simulink model "ANN_and_Fuzzy_NCD"  (R2024a)
settings: Solver=ode23  StartTime=0.0  StopTime=200  RelTol=1e-8  EnableMultiTasking=on
model workspace (MAT data in the model file):
  targetSettings3 : object (value not decoded)
values from neighbouring files (symbols this model uses):
  I = in1'    [ann_training.m]
  T = out1'    [ann_training.m]
undefined symbols (not defined in the file or in its folder): B, DL, DQ, m, M, magnitude, rg, W, xb, xg, Xudot, yb, yg, Yvdot, zb, zg, Zwdot
libraries: neural x270, simulink x28, fuzblock x3
(part 11 of 12)

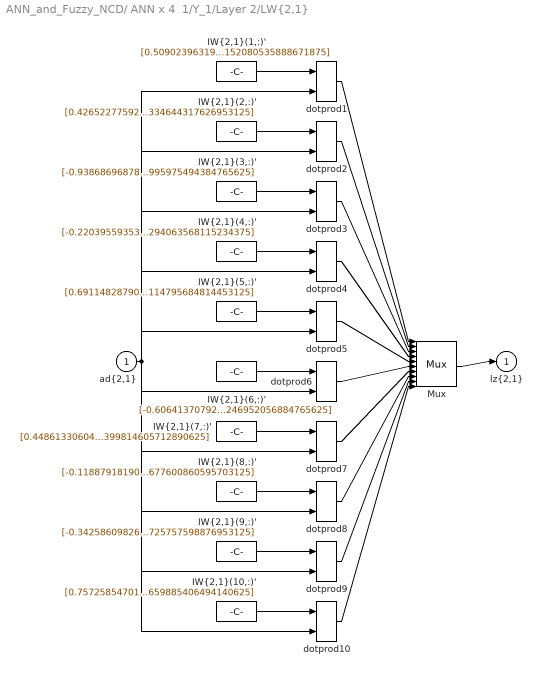
== system ANN_and_Fuzzy_NCD/ ANN x 4  1/Y_1/Layer 2/LW{2,1} ==
  "ad{2,1}" : Inport  PortDimensions=20
      mask Display: e = 0.06;c1 = [120 230 180]/255;c2 = ([120 230 180]+0)/(256+128);c3 = ([120 230 180]+128)/(256+128);patch([0 1 1 0],[0 0 1 1],c1);patch([0 1 1 1-e 1-e 0+e],[0 0 1 1-e 0+e 0+e],c2);patch([0 0 1 1-e 0+e 0+e],[0 1 1 1-e 1-e 0+e],c3);plot([0 1 1 0 0],[0 0 1 1 0]);
  "IW{2,1}(1,:)'" : Constant  Value=[0.5090239631979407430861783723230473697185516357421875;0.11160391846070348564889940234934329055249691009521484375;-0.60838467523272410364398865567636676132678985595703125;-0.45293416178246503900339803294627927243709564208984375;0.311166634755049076321853362969704903662204742431640625;0.330355832861899789687498696366674266755580902099609375;-0.57422288061641513223776200902648270130157470703125;-0.2838835075137227104136172783910296857357025146484375;-0.428001029373137054090392439320567063987255096435546875;0.62000342652741713411757018548087216913700103759765625;0.74336850402159060369200460627325810492038726806640625;-0.01139508661315961901561166769170085899531841278076171875;-0.61400475923319619564466620431630872189998626708984375;-0.05991076251349496117892812208083341829478740692138671875;0.84943975721566922221228423950378783047199249267578125;0.558146672456232284531552068074233829975128173828125;-0.042015831108889532818917444956241524778306484222412109375;0.460089284343286164524755577076575718820095062255859375;0.1646087842077264273843439923439291305840015411376953125;1.066820046479761696645027768681757152080535888671875]
      mask Display: e = 0.06;c1 = [120 150 230]/255;c2 = ([120 150 230]+0)/383;c3 = ([120 150 230]+128)/383;patch([0 1 1 0],[0 0 1 1],c1);patch([0 1 1 1-e 1-e 0+e],[0 0 1 1-e 0+e 0+e],c2);patch([0 0 1 1-e 0+e 0+e],[0 1 1 1-e 1-e 0+e],c3);plot([0 1 1 0 0],[0 0 1 1 0]);disp('weights');
  "IW{2,1}(10,:)'" : Constant  Value=[0.75725854701721961870219956836081109941005706787109375;0.74786484659251584172778848369489423930644989013671875;-0.37330720116505722305788594894693233072757720947265625;-0.25560543970363325261274667354882694780826568603515625;-0.3955234726214145180023251668899320065975189208984375;-0.1170710839775310485588732944961520843207836151123046875;0.130515477526785550477228525778627954423427581787109375;0.2277678588107421575603694918754626996815204620361328125;0.33980433602491155742342243684106506407260894775390625;-0.5489951844676215220175663489499129354953765869140625;0.7317112584413199005695105370250530540943145751953125;-0.42224791132812555805031706768204458057880401611328125;-0.11131793040447192366659834306119591929018497467041015625;-0.24585736991511353277672924377839080989360809326171875;-0.5961164816487041218096010197768919169902801513671875;-0.03003556254240373479813541734984028153121471405029296875;0.08420958263756218864504177190610789693892002105712890625;0.9050366596150227760375628349720500409603118896484375;0.46753348003908323793353929431759752333164215087890625;-0.039178527082161240802093971069552935659885406494140625]
      mask Display: e = 0.06;c1 = [120 150 230]/255;c2 = ([120 150 230]+0)/383;c3 = ([120 150 230]+128)/383;patch([0 1 1 0],[0 0 1 1],c1);patch([0 1 1 1-e 1-e 0+e],[0 0 1 1-e 0+e 0+e],c2);patch([0 0 1 1-e 0+e 0+e],[0 1 1 1-e 1-e 0+e],c3);plot([0 1 1 0 0],[0 0 1 1 0]);disp('weights');
  "IW{2,1}(2,:)'" : Constant  Value=[0.426522775921342967020422065616003237664699554443359375;0.11669002064379037364449942515420843847095966339111328125;-0.09094231709906390459519087698936345987021923065185546875;0.567514248708034241275299791595898568630218505859375;0.2537304330577907496291345523786731064319610595703125;-1.2920604784385449903538756188936531543731689453125;0.3414812039848078573101020083413459360599517822265625;0.263963170000102831380672796512953937053680419921875;-1.09849856655470023980569749255664646625518798828125;0.9864726214973646989392364048399031162261962890625;0.003132022306092559216228465857057017274200916290283203125;0.31270444346332448848357898896210826933383941650390625;-0.25315824125565578039953607003553770482540130615234375;-0.69773460760423111626238323879078961908817291259765625;-0.07611461049244357124354820598455262370407581329345703125;0.89021133988713707640982875091140158474445343017578125;0.6226655353392629432818239365587942302227020263671875;0.59260455755274688005584948768955655395984649658203125;-0.409387777619778514548443126841448247432708740234375;0.5890538696326192980023961354163475334644317626953125]
      mask Display: e = 0.06;c1 = [120 150 230]/255;c2 = ([120 150 230]+0)/383;c3 = ([120 150 230]+128)/383;patch([0 1 1 0],[0 0 1 1],c1);patch([0 1 1 1-e 1-e 0+e],[0 0 1 1-e 0+e 0+e],c2);patch([0 0 1 1-e 0+e 0+e],[0 1 1 1-e 1-e 0+e],c3);plot([0 1 1 0 0],[0 0 1 1 0]);disp('weights');
  "IW{2,1}(3,:)'" : Constant  Value=[-0.93868696878192781074545791852870024740695953369140625;-0.6377553662566040060255545540712773799896240234375;0.86418031487382329647317646958981640636920928955078125;1.0260293267344493539638961010496132075786590576171875;-0.58952068410571223378013883120729587972164154052734375;0.0992184017356094738460114967892877757549285888671875;0.62408971093074072644668603970785625278949737548828125;0.1697386682494127219111845761290169321000576019287109375;-1.1731596069625862543972516505164094269275665283203125;0.76298716435795699286614990342059172689914703369140625;-0.24277211963838796204839809433906339108943939208984375;-1.197372360644966438059100255486555397510528564453125;0.0712172363293012422591488075340748764574527740478515625;0.631562196722546875804482624516822397708892822265625;-0.192844601384166980384549106020131148397922515869140625;-0.1418385019727086138185967456593061797320842742919921875;0.386434553732358854194472996823606081306934356689453125;0.883931218735329427005353863933123648166656494140625;0.83856934978820907300445242071873508393764495849609375;1.8159130409844428388765891213552094995975494384765625]
      mask Display: e = 0.06;c1 = [120 150 230]/255;c2 = ([120 150 230]+0)/383;c3 = ([120 150 230]+128)/383;patch([0 1 1 0],[0 0 1 1],c1);patch([0 1 1 1-e 1-e 0+e],[0 0 1 1-e 0+e 0+e],c2);patch([0 0 1 1-e 0+e 0+e],[0 1 1 1-e 1-e 0+e],c3);plot([0 1 1 0 0],[0 0 1 1 0]);disp('weights');
  "IW{2,1}(4,:)'" : Constant  Value=[-0.22039559353873261482448242531972937285900115966796875;-0.2045148569053286402574798330533667467534542083740234375;-0.486566430678849914936989762281882576644420623779296875;-0.07025821021501608976134178874417557381093502044677734375;-0.658874386397240385804252582602202892303466796875;0.269798175500027159756655237288214266300201416015625;-0.1315210626537921811962661422512610442936420440673828125;-0.50169234000809359574901691303239203989505767822265625;2.141580948732917821786259082728065550327301025390625;0.37679791717396271533147000809549354016780853271484375;0.30916188174127656740353131681331433355808258056640625;-0.767499015164006426203968658228404819965362548828125;0.8980414488971601993938520536175929009914398193359375;-0.63991664257674429894251488804002292454242706298828125;-0.54821013988044364761975657529546879231929779052734375;0.52885732193772228004746693841298110783100128173828125;0.1540261738452853579328660771352588199079036712646484375;0.01847479725367588698770049404629389755427837371826171875;-0.333797443500849888575743307228549383580684661865234375;0.026821807331764944970498021348248585127294063568115234375]
      mask Display: e = 0.06;c1 = [120 150 230]/255;c2 = ([120 150 230]+0)/383;c3 = ([120 150 230]+128)/383;patch([0 1 1 0],[0 0 1 1],c1);patch([0 1 1 1-e 1-e 0+e],[0 0 1 1-e 0+e 0+e],c2);patch([0 0 1 1-e 0+e 0+e],[0 1 1 1-e 1-e 0+e],c3);plot([0 1 1 0 0],[0 0 1 1 0]);disp('weights');
  "IW{2,1}(5,:)'" : Constant  Value=[0.69114828790033266958658941803150810301303863525390625;0.55435534445943213111007707993849180638790130615234375;-0.9176208324668231330889511809800751507282257080078125;-0.10491305465673463059861347801415831781923770904541015625;-0.05473083756133391430953594181119115091860294342041015625;-0.27525707289210676886881401514983735978603363037109375;-0.0745176702560048642709489286062307655811309814453125;0.7894568146855700518926823860965669155120849609375;-1.68541642068066277460047786007635295391082763671875;-0.314903937294579494565738286837586201727390289306640625;0.1435542443257350198049238088060519658029079437255859375;-0.01012709573370276262826994440047201351262629032135009765625;0.16378713151763435451613304394413717091083526611328125;-0.361346282484408087842808754430734552443027496337890625;-0.03471757844671798098890036499142297543585300445556640625;-0.1938551744629932738206434805761091411113739013671875;-1.0324162610677387608149047082406468689441680908203125;-0.363503597064038341812874932656995952129364013671875;-0.4326961798445900786447282371227629482746124267578125;-0.65375618486997399969595790025778114795684814453125]
      mask Display: e = 0.06;c1 = [120 150 230]/255;c2 = ([120 150 230]+0)/383;c3 = ([120 150 230]+128)/383;patch([0 1 1 0],[0 0 1 1],c1);patch([0 1 1 1-e 1-e 0+e],[0 0 1 1-e 0+e 0+e],c2);patch([0 0 1 1-e 0+e 0+e],[0 1 1 1-e 1-e 0+e],c3);plot([0 1 1 0 0],[0 0 1 1 0]);disp('weights');
  "IW{2,1}(6,:)'" : Constant  Value=[-0.6064137079235631944129636394791305065155029296875;-0.70430664427252132053780542264576070010662078857421875;1.128267088531079931357226087129674851894378662109375;-0.01443760284603235431732937144033712684176862239837646484375;-0.1665820411319823557416697212829603813588619232177734375;-0.5448969322325221131819716902100481092929840087890625;0.1500632983600085623709929905089666135609149932861328125;0.491239762856461814610753435772494412958621978759765625;1.34531361537262217353827509214170277118682861328125;-0.65877809908486562040508260906790383160114288330078125;-0.2179297474681796409345935217061196453869342803955078125;-0.33324003089934317589637657874845899641513824462890625;0.331240335532091478842886544953216798603534698486328125;-0.140788452060973512391939266308327205479145050048828125;0.470179717315354850359909733015228994190692901611328125;0.32670818751247054922970391999115236103534698486328125;-0.30544754941956397953362056796322576701641082763671875;-0.179740446791701480311331806660746224224567413330078125;-0.53222231123358465509909365209750831127166748046875;-0.4198763573104165036653512288467027246952056884765625]
      mask Display: e = 0.06;c1 = [120 150 230]/255;c2 = ([120 150 230]+0)/383;c3 = ([120 150 230]+128)/383;patch([0 1 1 0],[0 0 1 1],c1);patch([0 1 1 1-e 1-e 0+e],[0 0 1 1-e 0+e 0+e],c2);patch([0 0 1 1-e 0+e 0+e],[0 1 1 1-e 1-e 0+e],c3);plot([0 1 1 0 0],[0 0 1 1 0]);disp('weights');
  "IW{2,1}(7,:)'" : Constant  Value=[0.448613306043071202733329982947907410562038421630859375;-0.1822903414610920480587452630061306990683078765869140625;-0.2126563507677423359165658212077687494456768035888671875;-0.28907878885491478104796669867937453091144561767578125;-0.5546330576663585087970886888797394931316375732421875;0.0881391364579335034878937449320801533758640289306640625;-0.005256269492573631234300091108480046386830508708953857421875;-0.13134253211367508118456726151634939014911651611328125;0.07828790111291732134457532765736686997115612030029296875;0.17303125336206737205912986610201187431812286376953125;0.04399549925057953669860211221021017991006374359130859375;0.1570358748639592849638546567803132347762584686279296875;-0.17807543738489750584363946472876705229282379150390625;0.2247661710889533315249622091869241558015346527099609375;-0.10691750616299990073176928717657574452459812164306640625;0.10221326745057923712778347180574201047420501708984375;0.94604303586329352437900297445594333112239837646484375;-0.31025843146322407140047516804770566523075103759765625;0.35028098540476559907830278461915440857410430908203125;-0.039186964941104164561469502814361476339399814605712890625]
      mask Display: e = 0.06;c1 = [120 150 230]/255;c2 = ([120 150 230]+0)/383;c3 = ([120 150 230]+128)/383;patch([0 1 1 0],[0 0 1 1],c1);patch([0 1 1 1-e 1-e 0+e],[0 0 1 1-e 0+e 0+e],c2);patch([0 0 1 1-e 0+e 0+e],[0 1 1 1-e 1-e 0+e],c3);plot([0 1 1 0 0],[0 0 1 1 0]);disp('weights');
  "IW{2,1}(8,:)'" : Constant  Value=[-0.1188791819001266680810857678807224147021770477294921875;-0.5328985881442112049199977263924665749073028564453125;0.5259930043630609564075939488247968256473541259765625;-0.355545136520511118050080767716281116008758544921875;-0.436040224271254495125305084002320654690265655517578125;-0.38339149391564586455416474564117379486560821533203125;-0.485397555278109849030698796923388727009296417236328125;-0.53377520344499862492426700555370189249515533447265625;1.538462588979844003489461101708002388477325439453125;0.240654646945936523394493633531965315341949462890625;0.65460238834859796330789549756445921957492828369140625;0.216226396066736936685259706791839562356472015380859375;-0.284211662449685931175480391175369732081890106201171875;-0.41705775992225502246668611405766569077968597412109375;-0.56091006758118755470832184073515236377716064453125;-0.6274337920918444666540381149388849735260009765625;1.057837377776273957152852744911797344684600830078125;-0.425439205099200690174399142051697708666324615478515625;-0.341212462205700839401600887867971323430538177490234375;0.0115945042058083098990284298679398489184677600860595703125]
      mask Display: e = 0.06;c1 = [120 150 230]/255;c2 = ([120 150 230]+0)/383;c3 = ([120 150 230]+128)/383;patch([0 1 1 0],[0 0 1 1],c1);patch([0 1 1 1-e 1-e 0+e],[0 0 1 1-e 0+e 0+e],c2);patch([0 0 1 1-e 0+e 0+e],[0 1 1 1-e 1-e 0+e],c3);plot([0 1 1 0 0],[0 0 1 1 0]);disp('weights');
  "IW{2,1}(9,:)'" : Constant  Value=[-0.3425860982600339443848724840790964663028717041015625;0.317963370391335209408367745709256269037723541259765625;0.38600757975739430349904068862088024616241455078125;0.11942370995519570320286817377564148046076297760009765625;-0.135297761504829860967902277479879558086395263671875;0.3811740311196782915459380092215724289417266845703125;-0.09833512570032722222013177315602661110460758209228515625;0.09431607025873588179276651999316527508199214935302734375;0.108063697459556851132589372355141676962375640869140625;0.93226980443745766091723226054455153644084930419921875;-0.198985445557301410257622364952112548053264617919921875;0.07278341181556084726889110925185377709567546844482421875;0.66596047086168541628836692325421608984470367431640625;-0.27925246224251842885877294975216500461101531982421875;-0.31408901001109590378490565854008309543132781982421875;-0.70192808772125558913757004120270721614360809326171875;-1.3726680003553408671024271825444884598255157470703125;-0.7352673542920313831672274318407289683818817138671875;-0.2476548671200008711057449772852123714983463287353515625;1.0455333746920534299107430342701263725757598876953125]
      mask Display: e = 0.06;c1 = [120 150 230]/255;c2 = ([120 150 230]+0)/383;c3 = ([120 150 230]+128)/383;patch([0 1 1 0],[0 0 1 1],c1);patch([0 1 1 1-e 1-e 0+e],[0 0 1 1-e 0+e 0+e],c2);patch([0 0 1 1-e 0+e 0+e],[0 1 1 1-e 1-e 0+e],c3);plot([0 1 1 0 0],[0 0 1 1 0]);disp('weights');
  Mux : Mux  Inputs=10
      mask Display: e = 0.06;c1 = [120 150 230]/255;c2 = ([120 150 230]+0)/383;c3 = ([120 150 230]+128)/383;patch([0 1 1 0],[0 0 1 1],c1);patch([0 1 1 1-e 1-e 0+e],[0 0 1 1-e 0+e 0+e],c2);patch([0 0 1 1-e 0+e 0+e],[0 1 1 1-e 1-e 0+e],c3);plot([0 1 1 0 0],[0 0 1 1 0]);disp('Mux');
  dotprod{1..10} (10 alike) : neural/Weight Functions/dotprod
  "lz{2,1}" : Outport
      mask Display: e = 0.06;c1 = [120 230 180]/255;c2 = ([120 230 180]+0)/(256+128);c3 = ([120 230 180]+128)/(256+128);patch([0 1 1 0],[0 0 1 1],c1);patch([0 1 1 1-e 1-e 0+e],[0 0 1 1-e 0+e 0+e],c2);patch([0 0 1 1-e 0+e 0+e],[0 1 1 1-e 1-e 0+e],c3);plot([0 1 1 0 0],[0 0 1 1 0]);
  wires:
  "IW{2,1}(1,:)'"/1 -> dotprod1/1
  "ad{2,1}"/1 -> dotprod1/2, dotprod2/2, dotprod3/2, dotprod4/2, dotprod5/2, dotprod6/2, dotprod7/2, dotprod8/2, dotprod9/2, dotprod10/2
  dotprod1/1 -> Mux/1
  "IW{2,1}(2,:)'"/1 -> dotprod2/1
  dotprod2/1 -> Mux/2
  "IW{2,1}(3,:)'"/1 -> dotprod3/1
  dotprod3/1 -> Mux/3
  "IW{2,1}(4,:)'"/1 -> dotprod4/1
  dotprod4/1 -> Mux/4
  "IW{2,1}(5,:)'"/1 -> dotprod5/1
  dotprod5/1 -> Mux/5
  "IW{2,1}(6,:)'"/1 -> dotprod6/1
  dotprod6/1 -> Mux/6
  "IW{2,1}(7,:)'"/1 -> dotprod7/1
  dotprod7/1 -> Mux/7
  "IW{2,1}(8,:)'"/1 -> dotprod8/1
  dotprod8/1 -> Mux/8
  "IW{2,1}(9,:)'"/1 -> dotprod9/1
  dotprod9/1 -> Mux/9
  "IW{2,1}(10,:)'"/1 -> dotprod10/1
  dotprod10/1 -> Mux/10
  Mux/1 -> "lz{2,1}"/1

== system ANN_and_Fuzzy_NCD/ ANN x 4  1/Y_1/Layer 3/Delays 1 ==
  "p{3}" : Inport  PortDimensions=10
      mask Display: e = 0.06;c1 = [120 230 180]/255;c2 = ([120 230 180]+0)/(256+128);c3 = ([120 230 180]+128)/(256+128);patch([0 1 1 0],[0 0 1 1],c1);patch([0 1 1 1-e 1-e 0+e],[0 0 1 1-e 0+e 0+e],c2);patch([0 0 1 1-e 0+e 0+e],[0 1 1 1-e 1-e 0+e],c3);plot([0 1 1 0 0],[0 0 1 1 0]);
  mux : Mux  Inputs=1
      mask Display: e = 0.06;c1 = [120 150 230]/255;c2 = ([120 150 230]+0)/383;c3 = ([120 150 230]+128)/383;patch([0 1 1 0],[0 0 1 1],c1);patch([0 1 1 1-e 1-e 0+e],[0 0 1 1-e 0+e 0+e],c2);patch([0 0 1 1-e 0+e 0+e],[0 1 1 1-e 1-e 0+e],c3);plot([0 1 1 0 0],[0 0 1 1 0]);disp('Mux')
  "pd{3,2}" : Outport
      mask Display: e = 0.06;c1 = [120 230 180]/255;c2 = ([120 230 180]+0)/(256+128);c3 = ([120 230 180]+128)/(256+128);patch([0 1 1 0],[0 0 1 1],c1);patch([0 1 1 1-e 1-e 0+e],[0 0 1 1-e 0+e 0+e],c2);patch([0 0 1 1-e 0+e 0+e],[0 1 1 1-e 1-e 0+e],c3);plot([0 1 1 0 0],[0 0 1 1 0]);
  wires:
  "p{3}"/1 -> mux/1
  mux/1 -> "pd{3,2}"/1

== system ANN_and_Fuzzy_NCD/ ANN x 4  1/Y_1/Layer 3/LW{3,2} ==
  "ad{3,2}" : Inport  PortDimensions=10
      mask Display: e = 0.06;c1 = [120 230 180]/255;c2 = ([120 230 180]+0)/(256+128);c3 = ([120 230 180]+128)/(256+128);patch([0 1 1 0],[0 0 1 1],c1);patch([0 1 1 1-e 1-e 0+e],[0 0 1 1-e 0+e 0+e],c2);patch([0 0 1 1-e 0+e 0+e],[0 1 1 1-e 1-e 0+e],c3);plot([0 1 1 0 0],[0 0 1 1 0]);
  "IW{3,2}(1,:)'" : Constant  Value=[-0.112703050539125104734239357640035450458526611328125;0.0026845090711100434884006649127741184202022850513458251953125;-0.006133432667343429074702232384197486680932343006134033203125;0.1331845640688972542964307876900420524179935455322265625;0.0978135232567727275210245352354831993579864501953125;0.71146262583635844212182064438820816576480865478515625;-0.151075401259040287271773195243440568447113037109375;0.11540184957138906185480919930341769941151142120361328125;0.07846874545309991122454817968900897540152072906494140625;0.1909190666063294294918506466274266131222248077392578125]
      mask Display: e = 0.06;c1 = [120 150 230]/255;c2 = ([120 150 230]+0)/383;c3 = ([120 150 230]+128)/383;patch([0 1 1 0],[0 0 1 1],c1);patch([0 1 1 1-e 1-e 0+e],[0 0 1 1-e 0+e 0+e],c2);patch([0 0 1 1-e 0+e 0+e],[0 1 1 1-e 1-e 0+e],c3);plot([0 1 1 0 0],[0 0 1 1 0]);disp('weights');
  Mux : Mux  Inputs=1
      mask Display: e = 0.06;c1 = [120 150 230]/255;c2 = ([120 150 230]+0)/383;c3 = ([120 150 230]+128)/383;patch([0 1 1 0],[0 0 1 1],c1);patch([0 1 1 1-e 1-e 0+e],[0 0 1 1-e 0+e 0+e],c2);patch([0 0 1 1-e 0+e 0+e],[0 1 1 1-e 1-e 0+e],c3);plot([0 1 1 0 0],[0 0 1 1 0]);disp('Mux');
  dotprod1 : neural/Weight Functions/dotprod
  "lz{3,2}" : Outport
      mask Display: e = 0.06;c1 = [120 230 180]/255;c2 = ([120 230 180]+0)/(256+128);c3 = ([120 230 180]+128)/(256+128);patch([0 1 1 0],[0 0 1 1],c1);patch([0 1 1 1-e 1-e 0+e],[0 0 1 1-e 0+e 0+e],c2);patch([0 0 1 1-e 0+e 0+e],[0 1 1 1-e 1-e 0+e],c3);plot([0 1 1 0 0],[0 0 1 1 0]);
  wires:
  "IW{3,2}(1,:)'"/1 -> dotprod1/1
  "ad{3,2}"/1 -> dotprod1/2
  dotprod1/1 -> Mux/1
  Mux/1 -> "lz{3,2}"/1

== system ANN_and_Fuzzy_NCD/ ANN x 4  1/Z_1/Layer 1/Delays 1 ==
  "p{1}" : Inport  PortDimensions=2
      mask Display: e = 0.06;c1 = [120 230 180]/255;c2 = ([120 230 180]+0)/(256+128);c3 = ([120 230 180]+128)/(256+128);patch([0 1 1 0],[0 0 1 1],c1);patch([0 1 1 1-e 1-e 0+e],[0 0 1 1-e 0+e 0+e],c2);patch([0 0 1 1-e 0+e 0+e],[0 1 1 1-e 1-e 0+e],c3);plot([0 1 1 0 0],[0 0 1 1 0]);
  mux : Mux  Inputs=1
      mask Display: e = 0.06;c1 = [120 150 230]/255;c2 = ([120 150 230]+0)/383;c3 = ([120 150 230]+128)/383;patch([0 1 1 0],[0 0 1 1],c1);patch([0 1 1 1-e 1-e 0+e],[0 0 1 1-e 0+e 0+e],c2);patch([0 0 1 1-e 0+e 0+e],[0 1 1 1-e 1-e 0+e],c3);plot([0 1 1 0 0],[0 0 1 1 0]);disp('Mux')
  "pd{1,1}" : Outport
      mask Display: e = 0.06;c1 = [120 230 180]/255;c2 = ([120 230 180]+0)/(256+128);c3 = ([120 230 180]+128)/(256+128);patch([0 1 1 0],[0 0 1 1],c1);patch([0 1 1 1-e 1-e 0+e],[0 0 1 1-e 0+e 0+e],c2);patch([0 0 1 1-e 0+e 0+e],[0 1 1 1-e 1-e 0+e],c3);plot([0 1 1 0 0],[0 0 1 1 0]);
  wires:
  "p{1}"/1 -> mux/1
  mux/1 -> "pd{1,1}"/1

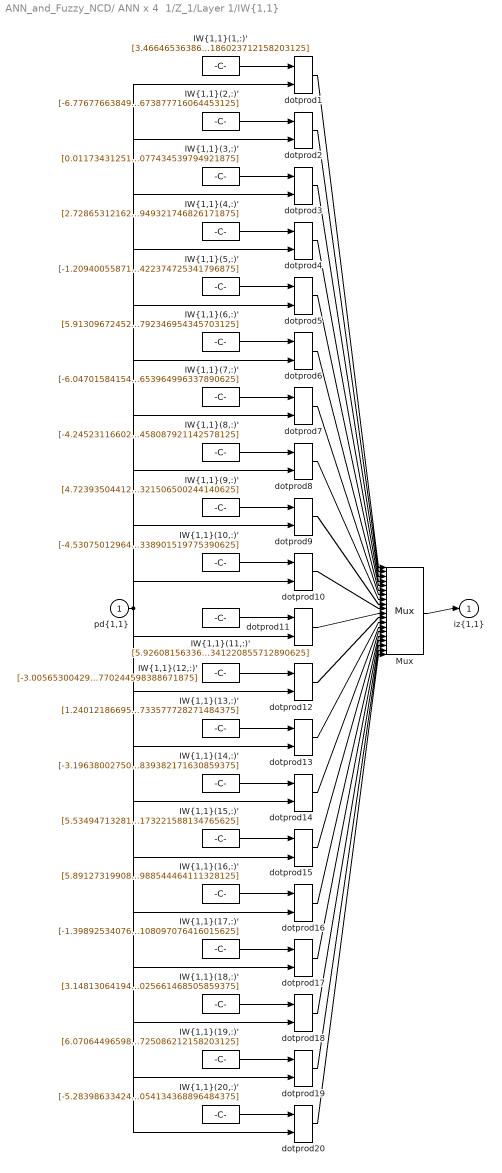
== system ANN_and_Fuzzy_NCD/ ANN x 4  1/Z_1/Layer 1/IW{1,1} ==
  "pd{1,1}" : Inport  PortDimensions=2
      mask Display: e = 0.06;c1 = [120 230 180]/255;c2 = ([120 230 180]+0)/(256+128);c3 = ([120 230 180]+128)/(256+128);patch([0 1 1 0],[0 0 1 1],c1);patch([0 1 1 1-e 1-e 0+e],[0 0 1 1-e 0+e 0+e],c2);patch([0 0 1 1-e 0+e 0+e],[0 1 1 1-e 1-e 0+e],c3);plot([0 1 1 0 0],[0 0 1 1 0]);
  "IW{1,1}(1,:)'" : Constant  Value=[3.466465363866880533549874598975293338298797607421875;-4.66357030032963582044658323866315186023712158203125]
      mask Display: e = 0.06;c1 = [120 150 230]/255;c2 = ([120 150 230]+0)/383;c3 = ([120 150 230]+128)/383;patch([0 1 1 0],[0 0 1 1],c1);patch([0 1 1 1-e 1-e 0+e],[0 0 1 1-e 0+e 0+e],c2);patch([0 0 1 1-e 0+e 0+e],[0 1 1 1-e 1-e 0+e],c3);plot([0 1 1 0 0],[0 0 1 1 0]);disp('Weights');
  "IW{1,1}(10,:)'" : Constant  Value=[-4.53075012964789092251294277957640588283538818359375;4.11465634782133182767438484006561338901519775390625]
      mask Display: e = 0.06;c1 = [120 150 230]/255;c2 = ([120 150 230]+0)/383;c3 = ([120 150 230]+128)/383;patch([0 1 1 0],[0 0 1 1],c1);patch([0 1 1 1-e 1-e 0+e],[0 0 1 1-e 0+e 0+e],c2);patch([0 0 1 1-e 0+e 0+e],[0 1 1 1-e 1-e 0+e],c3);plot([0 1 1 0 0],[0 0 1 1 0]);disp('Weights');
  "IW{1,1}(11,:)'" : Constant  Value=[5.926081563360074966340107494033873081207275390625;-2.050827965651885964604161927127279341220855712890625]
      mask Display: e = 0.06;c1 = [120 150 230]/255;c2 = ([120 150 230]+0)/383;c3 = ([120 150 230]+128)/383;patch([0 1 1 0],[0 0 1 1],c1);patch([0 1 1 1-e 1-e 0+e],[0 0 1 1-e 0+e 0+e],c2);patch([0 0 1 1-e 0+e 0+e],[0 1 1 1-e 1-e 0+e],c3);plot([0 1 1 0 0],[0 0 1 1 0]);disp('Weights');
  "IW{1,1}(12,:)'" : Constant  Value=[-3.005653004291876317921605732408352196216583251953125;5.56138941697332267466435951064340770244598388671875]
      mask Display: e = 0.06;c1 = [120 150 230]/255;c2 = ([120 150 230]+0)/383;c3 = ([120 150 230]+128)/383;patch([0 1 1 0],[0 0 1 1],c1);patch([0 1 1 1-e 1-e 0+e],[0 0 1 1-e 0+e 0+e],c2);patch([0 0 1 1-e 0+e 0+e],[0 1 1 1-e 1-e 0+e],c3);plot([0 1 1 0 0],[0 0 1 1 0]);disp('Weights');
  "IW{1,1}(13,:)'" : Constant  Value=[1.24012186695245674172838334925472736358642578125;-5.56429645265497896389206289313733577728271484375]
      mask Display: e = 0.06;c1 = [120 150 230]/255;c2 = ([120 150 230]+0)/383;c3 = ([120 150 230]+128)/383;patch([0 1 1 0],[0 0 1 1],c1);patch([0 1 1 1-e 1-e 0+e],[0 0 1 1-e 0+e 0+e],c2);patch([0 0 1 1-e 0+e 0+e],[0 1 1 1-e 1-e 0+e],c3);plot([0 1 1 0 0],[0 0 1 1 0]);disp('Weights');
  "IW{1,1}(14,:)'" : Constant  Value=[-3.196380027505041798718821155489422380924224853515625;-5.34177115724356266213135313591919839382171630859375]
      mask Display: e = 0.06;c1 = [120 150 230]/255;c2 = ([120 150 230]+0)/383;c3 = ([120 150 230]+128)/383;patch([0 1 1 0],[0 0 1 1],c1);patch([0 1 1 1-e 1-e 0+e],[0 0 1 1-e 0+e 0+e],c2);patch([0 0 1 1-e 0+e 0+e],[0 1 1 1-e 1-e 0+e],c3);plot([0 1 1 0 0],[0 0 1 1 0]);disp('Weights');
  "IW{1,1}(15,:)'" : Constant  Value=[5.5349471328160273486673759180121123790740966796875;1.734648888108174080713297371403314173221588134765625]
      mask Display: e = 0.06;c1 = [120 150 230]/255;c2 = ([120 150 230]+0)/383;c3 = ([120 150 230]+128)/383;patch([0 1 1 0],[0 0 1 1],c1);patch([0 1 1 1-e 1-e 0+e],[0 0 1 1-e 0+e 0+e],c2);patch([0 0 1 1-e 0+e 0+e],[0 1 1 1-e 1-e 0+e],c3);plot([0 1 1 0 0],[0 0 1 1 0]);disp('Weights');
  "IW{1,1}(16,:)'" : Constant  Value=[5.8912731990887845512361309374682605266571044921875;-1.8539195572739999295919233190943486988544464111328125]
      mask Display: e = 0.06;c1 = [120 150 230]/255;c2 = ([120 150 230]+0)/383;c3 = ([120 150 230]+128)/383;patch([0 1 1 0],[0 0 1 1],c1);patch([0 1 1 1-e 1-e 0+e],[0 0 1 1-e 0+e 0+e],c2);patch([0 0 1 1-e 0+e 0+e],[0 1 1 1-e 1-e 0+e],c3);plot([0 1 1 0 0],[0 0 1 1 0]);disp('Weights');
  "IW{1,1}(17,:)'" : Constant  Value=[-1.3989253407657382677342638999107293784618377685546875;-5.9319632349597473108815393061377108097076416015625]
      mask Display: e = 0.06;c1 = [120 150 230]/255;c2 = ([120 150 230]+0)/383;c3 = ([120 150 230]+128)/383;patch([0 1 1 0],[0 0 1 1],c1);patch([0 1 1 1-e 1-e 0+e],[0 0 1 1-e 0+e 0+e],c2);patch([0 0 1 1-e 0+e 0+e],[0 1 1 1-e 1-e 0+e],c3);plot([0 1 1 0 0],[0 0 1 1 0]);disp('Weights');
  "IW{1,1}(18,:)'" : Constant  Value=[3.148130641942957108625478213070891797542572021484375;-5.4125255982093616324846152565442025661468505859375]
      mask Display: e = 0.06;c1 = [120 150 230]/255;c2 = ([120 150 230]+0)/383;c3 = ([120 150 230]+128)/383;patch([0 1 1 0],[0 0 1 1],c1);patch([0 1 1 1-e 1-e 0+e],[0 0 1 1-e 0+e 0+e],c2);patch([0 0 1 1-e 0+e 0+e],[0 1 1 1-e 1-e 0+e],c3);plot([0 1 1 0 0],[0 0 1 1 0]);disp('Weights');
  "IW{1,1}(19,:)'" : Constant  Value=[6.070644965985930952001581317745149135589599609375;-0.97155605349458096231529680153471417725086212158203125]
      mask Display: e = 0.06;c1 = [120 150 230]/255;c2 = ([120 150 230]+0)/383;c3 = ([120 150 230]+128)/383;patch([0 1 1 0],[0 0 1 1],c1);patch([0 1 1 1-e 1-e 0+e],[0 0 1 1-e 0+e 0+e],c2);patch([0 0 1 1-e 0+e 0+e],[0 1 1 1-e 1-e 0+e],c3);plot([0 1 1 0 0],[0 0 1 1 0]);disp('Weights');
  "IW{1,1}(2,:)'" : Constant  Value=[-6.7767766384908814103482654900290071964263916015625;0.459789848930055644604664166763541288673877716064453125]
      mask Display: e = 0.06;c1 = [120 150 230]/255;c2 = ([120 150 230]+0)/383;c3 = ([120 150 230]+128)/383;patch([0 1 1 0],[0 0 1 1],c1);patch([0 1 1 1-e 1-e 0+e],[0 0 1 1-e 0+e 0+e],c2);patch([0 0 1 1-e 0+e 0+e],[0 1 1 1-e 1-e 0+e],c3);plot([0 1 1 0 0],[0 0 1 1 0]);disp('Weights');
  "IW{1,1}(20,:)'" : Constant  Value=[-5.28398633424957875348582092556171119213104248046875;-3.123211861841967529329622266232036054134368896484375]
      mask Display: e = 0.06;c1 = [120 150 230]/255;c2 = ([120 150 230]+0)/383;c3 = ([120 150 230]+128)/383;patch([0 1 1 0],[0 0 1 1],c1);patch([0 1 1 1-e 1-e 0+e],[0 0 1 1-e 0+e 0+e],c2);patch([0 0 1 1-e 0+e 0+e],[0 1 1 1-e 1-e 0+e],c3);plot([0 1 1 0 0],[0 0 1 1 0]);disp('Weights');
  "IW{1,1}(3,:)'" : Constant  Value=[0.0117343125153924650316827893448135000653564929962158203125;-6.07871661058124868048935240949504077434539794921875]
      mask Display: e = 0.06;c1 = [120 150 230]/255;c2 = ([120 150 230]+0)/383;c3 = ([120 150 230]+128)/383;patch([0 1 1 0],[0 0 1 1],c1);patch([0 1 1 1-e 1-e 0+e],[0 0 1 1-e 0+e 0+e],c2);patch([0 0 1 1-e 0+e 0+e],[0 1 1 1-e 1-e 0+e],c3);plot([0 1 1 0 0],[0 0 1 1 0]);disp('Weights');
  "IW{1,1}(4,:)'" : Constant  Value=[2.72865312162343709445622152998112142086029052734375;-2.940536892551005365703531424514949321746826171875]
      mask Display: e = 0.06;c1 = [120 150 230]/255;c2 = ([120 150 230]+0)/383;c3 = ([120 150 230]+128)/383;patch([0 1 1 0],[0 0 1 1],c1);patch([0 1 1 1-e 1-e 0+e],[0 0 1 1-e 0+e 0+e],c2);patch([0 0 1 1-e 0+e 0+e],[0 1 1 1-e 1-e 0+e],c3);plot([0 1 1 0 0],[0 0 1 1 0]);disp('Weights');
  "IW{1,1}(5,:)'" : Constant  Value=[-1.2094005587146410274357322123250924050807952880859375;-6.35487306582990907344310471671633422374725341796875]
      mask Display: e = 0.06;c1 = [120 150 230]/255;c2 = ([120 150 230]+0)/383;c3 = ([120 150 230]+128)/383;patch([0 1 1 0],[0 0 1 1],c1);patch([0 1 1 1-e 1-e 0+e],[0 0 1 1-e 0+e 0+e],c2);patch([0 0 1 1-e 0+e 0+e],[0 1 1 1-e 1-e 0+e],c3);plot([0 1 1 0 0],[0 0 1 1 0]);disp('Weights');
  "IW{1,1}(6,:)'" : Constant  Value=[5.91309672452974321998908635578118264675140380859375;-1.5680826906446097002145734222722239792346954345703125]
      mask Display: e = 0.06;c1 = [120 150 230]/255;c2 = ([120 150 230]+0)/383;c3 = ([120 150 230]+128)/383;patch([0 1 1 0],[0 0 1 1],c1);patch([0 1 1 1-e 1-e 0+e],[0 0 1 1-e 0+e 0+e],c2);patch([0 0 1 1-e 0+e 0+e],[0 1 1 1-e 1-e 0+e],c3);plot([0 1 1 0 0],[0 0 1 1 0]);disp('Weights');
  "IW{1,1}(7,:)'" : Constant  Value=[-6.04701584154958027284010313451290130615234375;-0.96931444603444882890386224971734918653964996337890625]
      mask Display: e = 0.06;c1 = [120 150 230]/255;c2 = ([120 150 230]+0)/383;c3 = ([120 150 230]+128)/383;patch([0 1 1 0],[0 0 1 1],c1);patch([0 1 1 1-e 1-e 0+e],[0 0 1 1-e 0+e 0+e],c2);patch([0 0 1 1-e 0+e 0+e],[0 1 1 1-e 1-e 0+e],c3);plot([0 1 1 0 0],[0 0 1 1 0]);disp('Weights');
  "IW{1,1}(8,:)'" : Constant  Value=[-4.24523116602744199354901866172440350055694580078125;5.063686262043830765833263285458087921142578125]
      mask Display: e = 0.06;c1 = [120 150 230]/255;c2 = ([120 150 230]+0)/383;c3 = ([120 150 230]+128)/383;patch([0 1 1 0],[0 0 1 1],c1);patch([0 1 1 1-e 1-e 0+e],[0 0 1 1-e 0+e 0+e],c2);patch([0 0 1 1-e 0+e 0+e],[0 1 1 1-e 1-e 0+e],c3);plot([0 1 1 0 0],[0 0 1 1 0]);disp('Weights');
  "IW{1,1}(9,:)'" : Constant  Value=[4.7239350441259375656954944133758544921875;4.1236383353300940513008754351176321506500244140625]
      mask Display: e = 0.06;c1 = [120 150 230]/255;c2 = ([120 150 230]+0)/383;c3 = ([120 150 230]+128)/383;patch([0 1 1 0],[0 0 1 1],c1);patch([0 1 1 1-e 1-e 0+e],[0 0 1 1-e 0+e 0+e],c2);patch([0 0 1 1-e 0+e 0+e],[0 1 1 1-e 1-e 0+e],c3);plot([0 1 1 0 0],[0 0 1 1 0]);disp('Weights');
  Mux : Mux  Inputs=20
      mask Display: e = 0.06;c1 = [120 150 230]/255;c2 = ([120 150 230]+0)/383;c3 = ([120 150 230]+128)/383;patch([0 1 1 0],[0 0 1 1],c1);patch([0 1 1 1-e 1-e 0+e],[0 0 1 1-e 0+e 0+e],c2);patch([0 0 1 1-e 0+e 0+e],[0 1 1 1-e 1-e 0+e],c3);plot([0 1 1 0 0],[0 0 1 1 0]);disp('Mux');
  dotprod{1..20} (20 alike) : neural/Weight Functions/dotprod
  "iz{1,1}" : Outport
      mask Display: e = 0.06;c1 = [120 230 180]/255;c2 = ([120 230 180]+0)/(256+128);c3 = ([120 230 180]+128)/(256+128);patch([0 1 1 0],[0 0 1 1],c1);patch([0 1 1 1-e 1-e 0+e],[0 0 1 1-e 0+e 0+e],c2);patch([0 0 1 1-e 0+e 0+e],[0 1 1 1-e 1-e 0+e],c3);plot([0 1 1 0 0],[0 0 1 1 0]);
  wires:
  "IW{1,1}(1,:)'"/1 -> dotprod1/1
  "pd{1,1}"/1 -> dotprod1/2, dotprod2/2, dotprod3/2, dotprod4/2, dotprod5/2, dotprod6/2, dotprod7/2, dotprod8/2, dotprod9/2, dotprod10/2, dotprod11/2, dotprod12/2, dotprod13/2, dotprod14/2, dotprod15/2, dotprod16/2, dotprod17/2, dotprod18/2, dotprod19/2, dotprod20/2
  dotprod1/1 -> Mux/1
  "IW{1,1}(2,:)'"/1 -> dotprod2/1
  dotprod2/1 -> Mux/2
  "IW{1,1}(3,:)'"/1 -> dotprod3/1
  dotprod3/1 -> Mux/3
  "IW{1,1}(4,:)'"/1 -> dotprod4/1
  dotprod4/1 -> Mux/4
  "IW{1,1}(5,:)'"/1 -> dotprod5/1
  dotprod5/1 -> Mux/5
  "IW{1,1}(6,:)'"/1 -> dotprod6/1
  dotprod6/1 -> Mux/6
  "IW{1,1}(7,:)'"/1 -> dotprod7/1
  dotprod7/1 -> Mux/7
  "IW{1,1}(8,:)'"/1 -> dotprod8/1
  dotprod8/1 -> Mux/8
  "IW{1,1}(9,:)'"/1 -> dotprod9/1
  dotprod9/1 -> Mux/9
  "IW{1,1}(10,:)'"/1 -> dotprod10/1
  dotprod10/1 -> Mux/10
  "IW{1,1}(11,:)'"/1 -> dotprod11/1
  dotprod11/1 -> Mux/11
  "IW{1,1}(12,:)'"/1 -> dotprod12/1
  dotprod12/1 -> Mux/12
  "IW{1,1}(13,:)'"/1 -> dotprod13/1
  dotprod13/1 -> Mux/13
  "IW{1,1}(14,:)'"/1 -> dotprod14/1
  dotprod14/1 -> Mux/14
  "IW{1,1}(15,:)'"/1 -> dotprod15/1
  dotprod15/1 -> Mux/15
  "IW{1,1}(16,:)'"/1 -> dotprod16/1
  dotprod16/1 -> Mux/16
  "IW{1,1}(17,:)'"/1 -> dotprod17/1
  dotprod17/1 -> Mux/17
  "IW{1,1}(18,:)'"/1 -> dotprod18/1
  dotprod18/1 -> Mux/18
  "IW{1,1}(19,:)'"/1 -> dotprod19/1
  dotprod19/1 -> Mux/19
  "IW{1,1}(20,:)'"/1 -> dotprod20/1
  dotprod20/1 -> Mux/20
  Mux/1 -> "iz{1,1}"/1

== system ANN_and_Fuzzy_NCD/ ANN x 4  1/Z_1/Layer 2/Delays 1 ==
  "p{2}" : Inport  PortDimensions=20
      mask Display: e = 0.06;c1 = [120 230 180]/255;c2 = ([120 230 180]+0)/(256+128);c3 = ([120 230 180]+128)/(256+128);patch([0 1 1 0],[0 0 1 1],c1);patch([0 1 1 1-e 1-e 0+e],[0 0 1 1-e 0+e 0+e],c2);patch([0 0 1 1-e 0+e 0+e],[0 1 1 1-e 1-e 0+e],c3);plot([0 1 1 0 0],[0 0 1 1 0]);
  mux : Mux  Inputs=1
      mask Display: e = 0.06;c1 = [120 150 230]/255;c2 = ([120 150 230]+0)/383;c3 = ([120 150 230]+128)/383;patch([0 1 1 0],[0 0 1 1],c1);patch([0 1 1 1-e 1-e 0+e],[0 0 1 1-e 0+e 0+e],c2);patch([0 0 1 1-e 0+e 0+e],[0 1 1 1-e 1-e 0+e],c3);plot([0 1 1 0 0],[0 0 1 1 0]);disp('Mux')
  "pd{2,1}" : Outport
      mask Display: e = 0.06;c1 = [120 230 180]/255;c2 = ([120 230 180]+0)/(256+128);c3 = ([120 230 180]+128)/(256+128);patch([0 1 1 0],[0 0 1 1],c1);patch([0 1 1 1-e 1-e 0+e],[0 0 1 1-e 0+e 0+e],c2);patch([0 0 1 1-e 0+e 0+e],[0 1 1 1-e 1-e 0+e],c3);plot([0 1 1 0 0],[0 0 1 1 0]);
  wires:
  "p{2}"/1 -> mux/1
  mux/1 -> "pd{2,1}"/1

== system ANN_and_Fuzzy_NCD/ ANN x 4  1/Z_1/Layer 2/LW{2,1} ==
  "ad{2,1}" : Inport  PortDimensions=20
      mask Display: e = 0.06;c1 = [120 230 180]/255;c2 = ([120 230 180]+0)/(256+128);c3 = ([120 230 180]+128)/(256+128);patch([0 1 1 0],[0 0 1 1],c1);patch([0 1 1 1-e 1-e 0+e],[0 0 1 1-e 0+e 0+e],c2);patch([0 0 1 1-e 0+e 0+e],[0 1 1 1-e 1-e 0+e],c3);plot([0 1 1 0 0],[0 0 1 1 0]);
  "IW{2,1}(1,:)'" : Constant  Value=[0.09390966812574012834158310170096228830516338348388671875;0.282170580794637138044578250628546811640262603759765625;-0.6879637650961194506038509643985889852046966552734375;0.08181124006185656882816914503564476035535335540771484375;-0.1741415527072056601554095323081128299236297607421875;-0.619267410036138610252010039403103291988372802734375;0.518631743651294829788866991293616592884063720703125;-0.5444985788617529021138352618436329066753387451171875;-0.53556259687692142623660629396908916532993316650390625;0.04276024256734010930980360853936872445046901702880859375;0.177524924143742601767570477022673003375530242919921875;0.334462762012160019775564023802871815860271453857421875;-0.206080971401598145309463916419190354645252227783203125;0.5878188864336892915929411174147389829158782958984375;-0.016641794532322264077439655238777049817144870758056640625;0.00653487196635476989825530580446866224519908428192138671875;-0.48598829757315409327844690778874792158603668212890625;0.41197335372927923469177358128945343196392059326171875;0.488547097211347869372133345677866600453853607177734375;0.28810844413750291703735229020821861922740936279296875]
      mask Display: e = 0.06;c1 = [120 150 230]/255;c2 = ([120 150 230]+0)/383;c3 = ([120 150 230]+128)/383;patch([0 1 1 0],[0 0 1 1],c1);patch([0 1 1 1-e 1-e 0+e],[0 0 1 1-e 0+e 0+e],c2);patch([0 0 1 1-e 0+e 0+e],[0 1 1 1-e 1-e 0+e],c3);plot([0 1 1 0 0],[0 0 1 1 0]);disp('weights');
  "IW{2,1}(10,:)'" : Constant  Value=[0.2813268925743399595518212663591839373111724853515625;0.1116123402451145441016677750667440705001354217529296875;0.29218758199615291193396160451811738312244415283203125;0.895359382063307673860208524274639785289764404296875;-0.71924337247869962741475546863512136042118072509765625;-0.231918596002188615035066732161794789135456085205078125;0.3773773582707036222672059011529199779033660888671875;-0.2405770848829871244589639900368638336658477783203125;-0.0913221340895489230859993767808191478252410888671875;-0.0160524819746029924483199380347286933101713657379150390625;0.2234660789061871655203361797248362563550472259521484375;0.5316102157457984755950519684120081365108489990234375;0.64291894169744268072719250994850881397724151611328125;-0.1505775339695645531623569013390806503593921661376953125;-0.379014252054569344974055411512381397187709808349609375;-0.312967533427033040016596032728557474911212921142578125;0.371768444519977314666192569347913376986980438232421875;-0.366623738642197050108251232813927344977855682373046875;0.297315940944873846607521272744634188711643218994140625;-0.03468494054867977960388003566549741663038730621337890625]
      mask Display: e = 0.06;c1 = [120 150 230]/255;c2 = ([120 150 230]+0)/383;c3 = ([120 150 230]+128)/383;patch([0 1 1 0],[0 0 1 1],c1);patch([0 1 1 1-e 1-e 0+e],[0 0 1 1-e 0+e 0+e],c2);patch([0 0 1 1-e 0+e 0+e],[0 1 1 1-e 1-e 0+e],c3);plot([0 1 1 0 0],[0 0 1 1 0]);disp('weights');
  "IW{2,1}(2,:)'" : Constant  Value=[-0.07431691891270240934996849091476178728044033050537109375;-0.14139917327275697278565758097101934254169464111328125;1.0940883266987935229508366319350898265838623046875;0.71553413824607725590709605967276729643344879150390625;-0.024338643017883077046548123689717613160610198974609375;-0.52302151489578607712616076241829432547092437744140625;0.1114025072475449407161107728825300000607967376708984375;0.67350602120265501415730113876634277403354644775390625;0.30561264119769460112507886151433922350406646728515625;-0.3847011149660606310618504721787758171558380126953125;0.09183197228038440795838681651730439625680446624755859375;0.428065300958234196126994675068999640643596649169921875;-0.350156427945300607884604460195987485349178314208984375;0.0513676414638426781511526542089995928108692169189453125;-0.142881307419454317564344592028646729886531829833984375;-0.873353819968668343420858946046791970729827880859375;0.8315185268680218566572648342116735875606536865234375;-0.006634255628174766904192605210255351266823709011077880859375;0.07322604338253209388387432454692316241562366485595703125;0.200077725398735972728303522671922110021114349365234375]
      mask Display: e = 0.06;c1 = [120 150 230]/255;c2 = ([120 150 230]+0)/383;c3 = ([120 150 230]+128)/383;patch([0 1 1 0],[0 0 1 1],c1);patch([0 1 1 1-e 1-e 0+e],[0 0 1 1-e 0+e 0+e],c2);patch([0 0 1 1-e 0+e 0+e],[0 1 1 1-e 1-e 0+e],c3);plot([0 1 1 0 0],[0 0 1 1 0]);disp('weights');
  "IW{2,1}(3,:)'" : Constant  Value=[-0.53676586635559875304579691146500408649444580078125;0.177518639318464732657076865507406182587146759033203125;-0.28069605338724901155700308663654141128063201904296875;-0.65658750023002399043292598435073159635066986083984375;1.080437178916152873853206983767449855804443359375;1.122341857259605557572967882151715457439422607421875;-0.8569683338574163311562870148918591439723968505859375;-1.2587357885084633490890837492770515382289886474609375;0.9644070741901040744181727859540842473506927490234375;-1.033089355318775659497987362556159496307373046875;0.46736220624287072578084689666866324841976165771484375;-1.0015055269160908490988504127017222344875335693359375;0.26579929093223564340320308474474586546421051025390625;-0.88698869021352688690740251331590116024017333984375;1.021731189975074283182721046614460647106170654296875;0.66422537280348226129689237495767883956432342529296875;-0.74551537661404243539919889371958561241626739501953125;1.1318443493252348108768501333543099462985992431640625;0.3362470490154099156399070125189609825611114501953125;-0.0237709904840943085646554067125180154107511043548583984375]
      mask Display: e = 0.06;c1 = [120 150 230]/255;c2 = ([120 150 230]+0)/383;c3 = ([120 150 230]+128)/383;patch([0 1 1 0],[0 0 1 1],c1);patch([0 1 1 1-e 1-e 0+e],[0 0 1 1-e 0+e 0+e],c2);patch([0 0 1 1-e 0+e 0+e],[0 1 1 1-e 1-e 0+e],c3);plot([0 1 1 0 0],[0 0 1 1 0]);disp('weights');
  "IW{2,1}(4,:)'" : Constant  Value=[0.46068407106841002818242714056395925581455230712890625;-0.2331366492595714212665569675664301030337810516357421875;0.5062552899396146610655478070839308202266693115234375;-0.320410795916360513491127903762389905750751495361328125;0.051923334155886201324303641513324691914021968841552734375;0.497465657239538894263120027972036041319370269775390625;0.4797926699780650228177591998246498405933380126953125;-0.0193502157536565265461003804148276685737073421478271484375;-0.848534978788809457483921505627222359180450439453125;0.53803609240071337271871243501664139330387115478515625;0.612399571666311981488206583890132606029510498046875;-0.07617743666550393089043069494437077082693576812744140625;0.11689282294705348463903504807603894732892513275146484375;-0.33472414654893423158199539102497510612010955810546875;-0.039972880603715198188918833466232172213494777679443359375;0.1616625654462170158520706308991066180169582366943359375;0.5014237194778701223185635171830654144287109375;0.367540794527864755902868409975781105458736419677734375;-0.313780834913472916891663544447510503232479095458984375;0.55837706942717246771934469506959430873394012451171875]
      mask Display: e = 0.06;c1 = [120 150 230]/255;c2 = ([120 150 230]+0)/383;c3 = ([120 150 230]+128)/383;patch([0 1 1 0],[0 0 1 1],c1);patch([0 1 1 1-e 1-e 0+e],[0 0 1 1-e 0+e 0+e],c2);patch([0 0 1 1-e 0+e 0+e],[0 1 1 1-e 1-e 0+e],c3);plot([0 1 1 0 0],[0 0 1 1 0]);disp('weights');
  "IW{2,1}(5,:)'" : Constant  Value=[-0.12589261053838429749163196902372874319553375244140625;0.08771179911247357907644328633978147991001605987548828125;-0.34160153534947779174757442888221703469753265380859375;0.43671996441230997998417251437786035239696502685546875;-0.19026139093429550452896137358038686215877532958984375;-0.471845850522515986025240408707759343087673187255859375;0.2361887280656885523821841843528090976178646087646484375;-0.229079597612783347759801699794479645788669586181640625;-0.236662752663826803090074690771871246397495269775390625;0.375494149495775531022445647977292537689208984375;-0.380661134546688983970597064399044029414653778076171875;0.6631594603090140704892974099493585526943206787109375;0.2272727820492925487894098068863968364894390106201171875;0.436065404367490694337305967565043829381465911865234375;0.078629920956626297989799923016107641160488128662109375;-0.2499852973307223613641525616912986151874065399169921875;0.1802086314523693444389351725476444698870182037353515625;0.44763549679784764290246812379336915910243988037109375;-0.40418088347513914104780496927560307085514068603515625;0.12411029725373208532079871702080708928406238555908203125]
      mask Display: e = 0.06;c1 = [120 150 230]/255;c2 = ([120 150 230]+0)/383;c3 = ([120 150 230]+128)/383;patch([0 1 1 0],[0 0 1 1],c1);patch([0 1 1 1-e 1-e 0+e],[0 0 1 1-e 0+e 0+e],c2);patch([0 0 1 1-e 0+e 0+e],[0 1 1 1-e 1-e 0+e],c3);plot([0 1 1 0 0],[0 0 1 1 0]);disp('weights');
  "IW{2,1}(6,:)'" : Constant  Value=[0.038345979614195176143898180498581496067345142364501953125;-0.1318791398876060505518381660294835455715656280517578125;0.55403005829233442636194695296580903232097625732421875;-0.02066133727786341467425046403150190599262714385986328125;0.339429393540805091067369403390330262482166290283203125;-0.2559145385822867435621219556196592748165130615234375;-0.432106040468774599272450132048106752336025238037109375;0.467819638327151288148542107592220418155193328857421875;0.0005985368636643854413359466803967734449543058872222900390625;-0.393400774719298740311757001109072007238864898681640625;-0.1579650395234692139556642587194801308214664459228515625;0.49446547843570820557346223722561262547969818115234375;0.41019660808221491965497307319310493767261505126953125;-0.296122301876966975697769157704897224903106689453125;0.1350228780584444010504086008950253017246723175048828125;0.477331939722515474766595389155554585158824920654296875;-0.369815266486423432912289399610017426311969757080078125;0.28208383832256433976226617232896387577056884765625;0.5043780241440753986381650975090451538562774658203125;-0.465011397164962481109995451333816163241863250732421875]
      mask Display: e = 0.06;c1 = [120 150 230]/255;c2 = ([120 150 230]+0)/383;c3 = ([120 150 230]+128)/383;patch([0 1 1 0],[0 0 1 1],c1);patch([0 1 1 1-e 1-e 0+e],[0 0 1 1-e 0+e 0+e],c2);patch([0 0 1 1-e 0+e 0+e],[0 1 1 1-e 1-e 0+e],c3);plot([0 1 1 0 0],[0 0 1 1 0]);disp('weights');
  "IW{2,1}(7,:)'" : Constant  Value=[-0.6632963042290718203020105647738091647624969482421875;0.92816678895914439539893692199257202446460723876953125;0.84427444459868450366002434748224914073944091796875;0.7454716761902397959005384109332226216793060302734375;0.9944579771594970196701979148201644420623779296875;0.71042421787458909232526593768852762877941131591796875;-1.0653998713148025156982612315914593636989593505859375;0.400692028627316398914359751870506443083286285400390625;-0.88778653297904874808210706760291941463947296142578125;-0.264599738495467862176013795760809443891048431396484375;-0.25676121400895823843057996782590635120868682861328125;0.05609538611639421079591016905396827496588230133056640625;0.270305279932320396962808217722340486943721771240234375;-0.1013965156265205502794657377307885326445102691650390625;0.173158865392192107268698464395129121840000152587890625;-0.31728880810445703186672972151427529752254486083984375;-0.375125587406057448003338095077197067439556121826171875;-0.1875403472037038554720567162803490646183490753173828125;0.032271670111766605215652958804639638401567935943603515625;0.53653616067539910972072902950458228588104248046875]
      mask Display: e = 0.06;c1 = [120 150 230]/255;c2 = ([120 150 230]+0)/383;c3 = ([120 150 230]+128)/383;patch([0 1 1 0],[0 0 1 1],c1);patch([0 1 1 1-e 1-e 0+e],[0 0 1 1-e 0+e 0+e],c2);patch([0 0 1 1-e 0+e 0+e],[0 1 1 1-e 1-e 0+e],c3);plot([0 1 1 0 0],[0 0 1 1 0]);disp('weights');
  "IW{2,1}(8,:)'" : Constant  Value=[-0.468853807016293255838235154442372731864452362060546875;0.046197533014600222767143122837296687066555023193359375;-0.2150942706046372887573880916534108109772205352783203125;-0.60524619826420522628040998824872076511383056640625;-0.1532347476681861497826986351356026716530323028564453125;-0.1545216076864319998396268829310429282486438751220703125;0.5324274450374577583033897099085152149200439453125;-0.54178288198241342232819306445890106260776519775390625;-0.369536978145258154793140192850842140614986419677734375;0.346168507596329166897675122527289204299449920654296875;-0.01879857644425679541466678301731008104979991912841796875;0.428104425748951855634771845871000550687313079833984375;-0.366638222650253364776062880991958081722259521484375;0.292592973699334513160152937416569329798221588134765625;-0.148005770727792473895334524058853276073932647705078125;-0.048644950419272518782332070941265556029975414276123046875;0.442290074747592132364815142864244990050792694091796875;-0.65660290188604164551833264340530149638652801513671875;-0.4295006586017340310945655801333487033843994140625;-0.026008928021298005628381133647053502500057220458984375]
      mask Display: e = 0.06;c1 = [120 150 230]/255;c2 = ([120 150 230]+0)/383;c3 = ([120 150 230]+128)/383;patch([0 1 1 0],[0 0 1 1],c1);patch([0 1 1 1-e 1-e 0+e],[0 0 1 1-e 0+e 0+e],c2);patch([0 0 1 1-e 0+e 0+e],[0 1 1 1-e 1-e 0+e],c3);plot([0 1 1 0 0],[0 0 1 1 0]);disp('weights');
  "IW{2,1}(9,:)'" : Constant  Value=[-0.84673256907712579621971826782100833952426910400390625;-0.034360010828392524573349220418094773776829242706298828125;0.6521905245978738552281583906733430922031402587890625;-0.07398303072464688934228860262010130099952220916748046875;0.50759829331218508929879362767678685486316680908203125;0.09687147546346015769547221907487255521118640899658203125;-0.11736408805743279992750416340641095302999019622802734375;0.51159801312223718294802665695897303521633148193359375;-0.53686004369026074645177004640572704374790191650390625;-0.09292888523912011533578692024093470536172389984130859375;0.11599975431695015715138907808068324811756610870361328125;0.3495883517078646196551972025190480053424835205078125;0.450128269946540149337721459232852794229984283447265625;0.2570304712350253151242895910399965941905975341796875;-0.54147390959565167012357278508716262876987457275390625;-0.29294797878476452890339487566961906850337982177734375;0.426392621527255155644553497040760703384876251220703125;-0.0883840073273914061946499032274005003273487091064453125;-0.570982573280862215625575117883272469043731689453125;-0.1263638293106170429336287952537531964480876922607421875]
      mask Display: e = 0.06;c1 = [120 150 230]/255;c2 = ([120 150 230]+0)/383;c3 = ([120 150 230]+128)/383;patch([0 1 1 0],[0 0 1 1],c1);patch([0 1 1 1-e 1-e 0+e],[0 0 1 1-e 0+e 0+e],c2);patch([0 0 1 1-e 0+e 0+e],[0 1 1 1-e 1-e 0+e],c3);plot([0 1 1 0 0],[0 0 1 1 0]);disp('weights');
  Mux : Mux  Inputs=10
      mask Display: e = 0.06;c1 = [120 150 230]/255;c2 = ([120 150 230]+0)/383;c3 = ([120 150 230]+128)/383;patch([0 1 1 0],[0 0 1 1],c1);patch([0 1 1 1-e 1-e 0+e],[0 0 1 1-e 0+e 0+e],c2);patch([0 0 1 1-e 0+e 0+e],[0 1 1 1-e 1-e 0+e],c3);plot([0 1 1 0 0],[0 0 1 1 0]);disp('Mux');
  dotprod{1..10} (10 alike) : neural/Weight Functions/dotprod
  "lz{2,1}" : Outport
      mask Display: e = 0.06;c1 = [120 230 180]/255;c2 = ([120 230 180]+0)/(256+128);c3 = ([120 230 180]+128)/(256+128);patch([0 1 1 0],[0 0 1 1],c1);patch([0 1 1 1-e 1-e 0+e],[0 0 1 1-e 0+e 0+e],c2);patch([0 0 1 1-e 0+e 0+e],[0 1 1 1-e 1-e 0+e],c3);plot([0 1 1 0 0],[0 0 1 1 0]);
  wires:
  "IW{2,1}(1,:)'"/1 -> dotprod1/1
  "ad{2,1}"/1 -> dotprod1/2, dotprod2/2, dotprod3/2, dotprod4/2, dotprod5/2, dotprod6/2, dotprod7/2, dotprod8/2, dotprod9/2, dotprod10/2
  dotprod1/1 -> Mux/1
  "IW{2,1}(2,:)'"/1 -> dotprod2/1
  dotprod2/1 -> Mux/2
  "IW{2,1}(3,:)'"/1 -> dotprod3/1
  dotprod3/1 -> Mux/3
  "IW{2,1}(4,:)'"/1 -> dotprod4/1
  dotprod4/1 -> Mux/4
  "IW{2,1}(5,:)'"/1 -> dotprod5/1
  dotprod5/1 -> Mux/5
  "IW{2,1}(6,:)'"/1 -> dotprod6/1
  dotprod6/1 -> Mux/6
  "IW{2,1}(7,:)'"/1 -> dotprod7/1
  dotprod7/1 -> Mux/7
  "IW{2,1}(8,:)'"/1 -> dotprod8/1
  dotprod8/1 -> Mux/8
  "IW{2,1}(9,:)'"/1 -> dotprod9/1
  dotprod9/1 -> Mux/9
  "IW{2,1}(10,:)'"/1 -> dotprod10/1
  dotprod10/1 -> Mux/10
  Mux/1 -> "lz{2,1}"/1
